simulink model "pwm_adc_sampling_timing"  (R2024b)
settings: Solver=FixedStepDiscrete  StartTime=0.0  StopTime=0  FixedStep=1  RelTol=1e-3
InitFcn:
  | model_file = get_param(bdroot, 'FileName');
  | model_dir = fileparts(model_file);
  | run(fullfile(model_dir, 'pwm_adc_sampling_params.m'));
values from neighbouring files (symbols this model uses):
  adc_fallback_ccr = pwm_half_arr    (= 2655)    [pwm_adc_sampling_params.m]
  adc_hold_last_on_fallback = 1    [pwm_adc_sampling_params.m]
  adc_margin_ccr = 140    [pwm_adc_sampling_params.m]
  adc_min_window_ccr = 320    [pwm_adc_sampling_params.m]
  adc_sample_max_ccr = pwm_arr - adc_margin_ccr    (= 5171)    [pwm_adc_sampling_params.m]
  adc_sample_min_ccr = adc_margin_ccr    (= 140)    [pwm_adc_sampling_params.m]
  pwm_arr = 5311    [pwm_adc_sampling_params.m]    (also in run_pwm_adc_sampling_timing_tests.m = local_param('pwm_arr'))
  pwm_half_arr = 2655    [pwm_adc_sampling_params.m]
  svpwm_max_ccr = pwm_arr - 20    (= 5291)    [pwm_adc_sampling_params.m]
  svpwm_min_ccr = 20    [pwm_adc_sampling_params.m]
  vbus = 24.0    (= 24)    [pwm_adc_sampling_params.m]
settings Model: Creator=10095  LastModifiedBy=10095

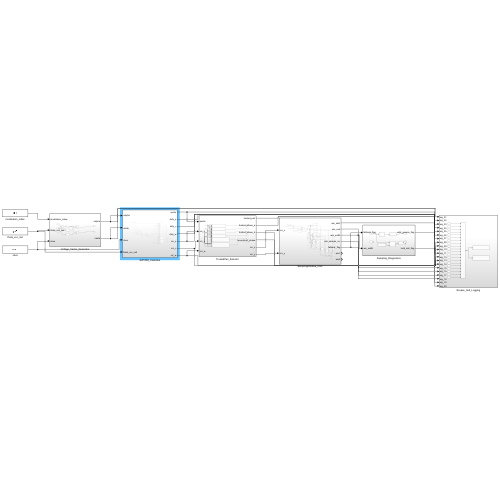
[thumbnail: Simulink's stored preview of the top-level diagram]
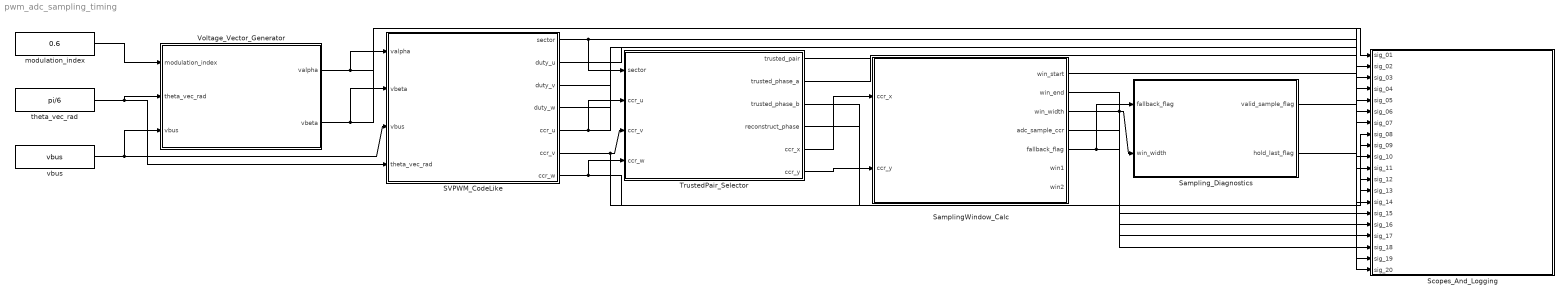
== system pwm_adc_sampling_timing ==
  SVPWM_CodeLike : Subsystem
  SamplingWindow_Calc : Subsystem
  Sampling_Diagnostics : Subsystem
  Scopes_And_Logging : Subsystem
  TrustedPair_Selector : Subsystem
  Voltage_Vector_Generator : Subsystem
  modulation_index : Constant  Value=0.6
  theta_vec_rad : Constant  Value=pi/6
  vbus : Constant  Value=vbus
  wires:
  modulation_index/1 -> Voltage_Vector_Generator/1(modulation_index)
  theta_vec_rad/1 -> Voltage_Vector_Generator/2(theta_vec_rad), SVPWM_CodeLike/4(theta_vec_rad)
  vbus/1 -> Voltage_Vector_Generator/3(vbus), SVPWM_CodeLike/3(vbus)
  Voltage_Vector_Generator/1(valpha) -> SVPWM_CodeLike/1(valpha), Scopes_And_Logging/1(sig_01)
  Voltage_Vector_Generator/2(vbeta) -> SVPWM_CodeLike/2(vbeta), Scopes_And_Logging/2(sig_02)
  SVPWM_CodeLike/1(sector) -> TrustedPair_Selector/1(sector), Scopes_And_Logging/3(sig_03)
  SVPWM_CodeLike/5(ccr_u) -> TrustedPair_Selector/2(ccr_u), Scopes_And_Logging/7(sig_07)
  SVPWM_CodeLike/6(ccr_v) -> TrustedPair_Selector/3(ccr_v), Scopes_And_Logging/8(sig_08)
  SVPWM_CodeLike/7(ccr_w) -> TrustedPair_Selector/4(ccr_w), Scopes_And_Logging/9(sig_09)
  TrustedPair_Selector/5(ccr_x) -> SamplingWindow_Calc/1(ccr_x)
  TrustedPair_Selector/6(ccr_y) -> SamplingWindow_Calc/2(ccr_y)
  SamplingWindow_Calc/5(fallback_flag) -> Sampling_Diagnostics/1(fallback_flag), Scopes_And_Logging/18(sig_18)
  SamplingWindow_Calc/3(win_width) -> Sampling_Diagnostics/2(win_width), Scopes_And_Logging/16(sig_16)
  SVPWM_CodeLike/2(duty_u) -> Scopes_And_Logging/4(sig_04)
  SVPWM_CodeLike/3(duty_v) -> Scopes_And_Logging/5(sig_05)
  SVPWM_CodeLike/4(duty_w) -> Scopes_And_Logging/6(sig_06)
  TrustedPair_Selector/1(trusted_pair) -> Scopes_And_Logging/10(sig_10)
  TrustedPair_Selector/2(trusted_phase_a) -> Scopes_And_Logging/11(sig_11)
  TrustedPair_Selector/3(trusted_phase_b) -> Scopes_And_Logging/12(sig_12)
  TrustedPair_Selector/4(reconstruct_phase) -> Scopes_And_Logging/13(sig_13)
  SamplingWindow_Calc/1(win_start) -> Scopes_And_Logging/14(sig_14)
  SamplingWindow_Calc/2(win_end) -> Scopes_And_Logging/15(sig_15)
  SamplingWindow_Calc/4(adc_sample_ccr) -> Scopes_And_Logging/17(sig_17)
  Sampling_Diagnostics/1(valid_sample_flag) -> Scopes_And_Logging/19(sig_19)
  Sampling_Diagnostics/2(hold_last_flag) -> Scopes_And_Logging/20(sig_20)

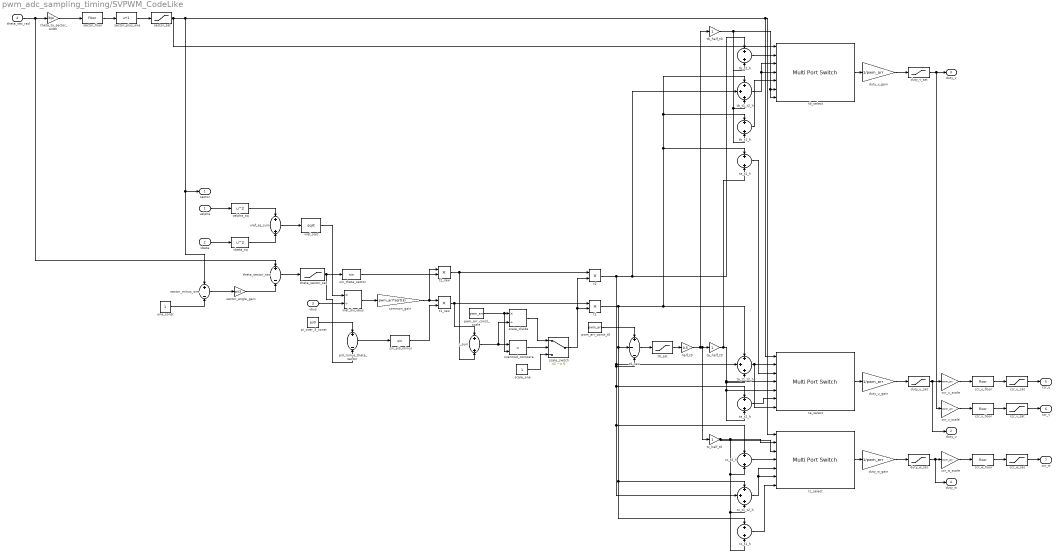
== system pwm_adc_sampling_timing/SVPWM_CodeLike ==
  valpha : Inport
  vbeta : Inport  Port=2
  vbus : Inport  Port=3
  theta_vec_rad : Inport  Port=4
  ccr_u_floor : Rounding
  ccr_u_sat : Saturate  UpperLimit=svpwm_max_ccr  LowerLimit=svpwm_min_ccr
  ccr_u_scale : Gain  Gain=pwm_arr
  ccr_v_floor : Rounding
  ccr_v_sat : Saturate  UpperLimit=svpwm_max_ccr  LowerLimit=svpwm_min_ccr
  ccr_v_scale : Gain  Gain=pwm_arr
  ccr_w_floor : Rounding
  ccr_w_sat : Saturate  UpperLimit=svpwm_max_ccr  LowerLimit=svpwm_min_ccr
  ccr_w_scale : Gain  Gain=pwm_arr
  common_gain : Gain  Gain=pwm_arr*sqrt(3)
  duty_u_gain : Gain  Gain=1/pwm_arr
  duty_u_sat : Saturate  UpperLimit=1  LowerLimit=0
  duty_v_gain : Gain  Gain=1/pwm_arr
  duty_v_sat : Saturate  UpperLimit=1  LowerLimit=0
  duty_w_gain : Gain  Gain=1/pwm_arr
  duty_w_sat : Saturate  UpperLimit=1  LowerLimit=0
  half_t0 : Gain  Gain=0.5
  one_const : Constant
  overmod_compare : RelationalOperator  Operator=>  OutDataTypeStr=boolean  RndMeth=Simplest  InputSameDT=off
  pi3_minus_theta_sector : Sum  Inputs=+-
  pi_over_3_const : Constant  Value=pi/3
  pwm_arr_const_scale : Constant  Value=pwm_arr
  pwm_arr_const_t0 : Constant  Value=pwm_arr
  scale_divide : Product  Inputs=*/
  scale_one : Constant
  scale_switch : Switch  Criteria=u2 ~= 0  SaturateOnIntegerOverflow=off  InputSameDT=off
  sector_angle_gain : Gain  Gain=pi/3
  sector_floor : Rounding
  sector_minus_one : Sum  Inputs=+-
  sector_plus_one : Bias  Bias=1  SaturateOnIntegerOverflow=off
  sector_sat : Saturate  UpperLimit=6  LowerLimit=1
  sin_pi3_minus : Trigonometry
  sin_theta_sector : Trigonometry
  t0_raw : Sum  Inputs=+--
  t0_sat : Saturate  UpperLimit=pwm_arr  LowerLimit=0
  t1 : Product
  t1_raw : Product
  t2 : Product
  t2_raw : Product
  t_sum : Sum
  ta_half_t0 : Gain
  ta_select : MultiPortSwitch  Inputs=6  SaturateOnIntegerOverflow=off  InputSameDT=off
  ta_t1_h : Sum
  ta_t1_t2_h : Sum  Inputs=+++
  ta_t2_h : Sum
  tb_half_t0 : Gain
  tb_select : MultiPortSwitch  Inputs=6  SaturateOnIntegerOverflow=off  InputSameDT=off
  tb_t1_h : Sum
  tb_t1_t2_h : Sum  Inputs=+++
  tb_t2_h : Sum
  tc_half_t0 : Gain
  tc_select : MultiPortSwitch  Inputs=6  SaturateOnIntegerOverflow=off  InputSameDT=off
  tc_t1_h : Sum
  tc_t1_t2_h : Sum  Inputs=+++
  tc_t2_h : Sum
  theta_sector_raw : Sum  Inputs=+-
  theta_sector_sat : Saturate  UpperLimit=pi/3  LowerLimit=0
  theta_to_sector_width : Gain  Gain=3/pi
  valpha_sq : Math  Operator=square
  vbeta_sq : Math  Operator=square
  vref_div_vbus : Product  Inputs=*/
  vref_sq_sum : Sum
  vref_sqrt : Math  Operator=sqrt
  sector : Outport
  duty_u : Outport  Port=2
  duty_v : Outport  Port=3
  duty_w : Outport  Port=4
  ccr_u : Outport  Port=5
  ccr_v : Outport  Port=6
  ccr_w : Outport  Port=7
  wires:
  theta_vec_rad/1 -> theta_to_sector_width/1, theta_sector_raw/1
  theta_to_sector_width/1 -> sector_floor/1
  sector_floor/1 -> sector_plus_one/1
  sector_sat/1 -> sector_minus_one/1, sector/1, ta_select/1, tc_select/1, tb_select/1
  sector_plus_one/1 -> sector_sat/1
  duty_v_gain/1 -> duty_v_sat/1
  one_const/1 -> sector_minus_one/2
  ta_t2_h/1 -> ta_select/6
  vbeta/1 -> vbeta_sq/1
  valpha/1 -> valpha_sq/1
  pi3_minus_theta_sector/1 -> sin_pi3_minus/1
  sector_minus_one/1 -> sector_angle_gain/1
  ccr_u_scale/1 -> ccr_u_floor/1
  valpha_sq/1 -> vref_sq_sum/1
  vbeta_sq/1 -> vref_sq_sum/2
  t0_sat/1 -> half_t0/1
  t0_raw/1 -> t0_sat/1
  sin_theta_sector/1 -> t2_raw/2
  sector_angle_gain/1 -> theta_sector_raw/2
  t1_raw/1 -> t1/1, t_sum/1
  vref_sq_sum/1 -> vref_sqrt/1
  ccr_v_floor/1 -> ccr_v_sat/1
  ta_half_t0/1 -> ta_t2_h/2, ta_select/5, ta_t1_t2_h/3, ta_select/4, ta_t1_h/2
  scale_switch/1 -> t1/2, t2/2
  theta_sector_raw/1 -> theta_sector_sat/1
  pwm_arr_const_scale/1 -> scale_divide/1, overmod_compare/2
  vref_sqrt/1 -> vref_div_vbus/1
  theta_sector_sat/1 -> pi3_minus_theta_sector/2, sin_theta_sector/1
  tc_select/1 -> duty_w_gain/1
  vbus/1 -> vref_div_vbus/2
  pi_over_3_const/1 -> pi3_minus_theta_sector/1
  vref_div_vbus/1 -> common_gain/1
  overmod_compare/1 -> scale_switch/2
  common_gain/1 -> t1_raw/1, t2_raw/1
  sin_pi3_minus/1 -> t1_raw/2
  ccr_w_sat/1 -> ccr_w/1
  t_sum/1 -> scale_divide/2, overmod_compare/1
  t2_raw/1 -> t_sum/2, t2/1
  scale_one/1 -> scale_switch/3
  scale_divide/1 -> scale_switch/1
  t2/1 -> tc_t2_h/1, tc_t1_t2_h/2, ta_t2_h/1, t0_raw/3, ta_t1_t2_h/2, tb_t2_h/1, tb_t1_t2_h/2
  tb_select/1 -> duty_v_gain/1
  t1/1 -> tc_t1_t2_h/1, tc_t1_h/1, t0_raw/2, tb_t1_h/1, tb_t1_t2_h/1, ta_t1_h/1, ta_t1_t2_h/1
  pwm_arr_const_t0/1 -> t0_raw/1
  ccr_w_scale/1 -> ccr_w_floor/1
  duty_w_sat/1 -> duty_w/1, ccr_w_scale/1
  duty_v_sat/1 -> duty_v/1, ccr_v_scale/1
  tb_t2_h/1 -> tb_select/2
  half_t0/1 -> tc_half_t0/1, ta_half_t0/1, tb_half_t0/1
  tb_half_t0/1 -> tb_t1_h/2, tb_t1_t2_h/3, tb_select/7, tb_select/6, tb_t2_h/2
  tc_half_t0/1 -> tc_t1_h/2, tc_t1_t2_h/3, tc_t2_h/2, tc_select/2, tc_select/3
  tb_t1_t2_h/1 -> tb_select/3, tb_select/4
  tb_t1_h/1 -> tb_select/5
  ta_t1_h/1 -> ta_select/3
  ta_t1_t2_h/1 -> ta_select/7, ta_select/2
  tc_t2_h/1 -> tc_select/4
  tc_t1_h/1 -> tc_select/7
  tc_t1_t2_h/1 -> tc_select/5, tc_select/6
  ta_select/1 -> duty_u_gain/1
  duty_u_gain/1 -> duty_u_sat/1
  duty_w_gain/1 -> duty_w_sat/1
  duty_u_sat/1 -> duty_u/1, ccr_u_scale/1
  ccr_v_scale/1 -> ccr_v_floor/1
  ccr_u_floor/1 -> ccr_u_sat/1
  ccr_w_floor/1 -> ccr_w_sat/1
  ccr_u_sat/1 -> ccr_u/1
  ccr_v_sat/1 -> ccr_v/1

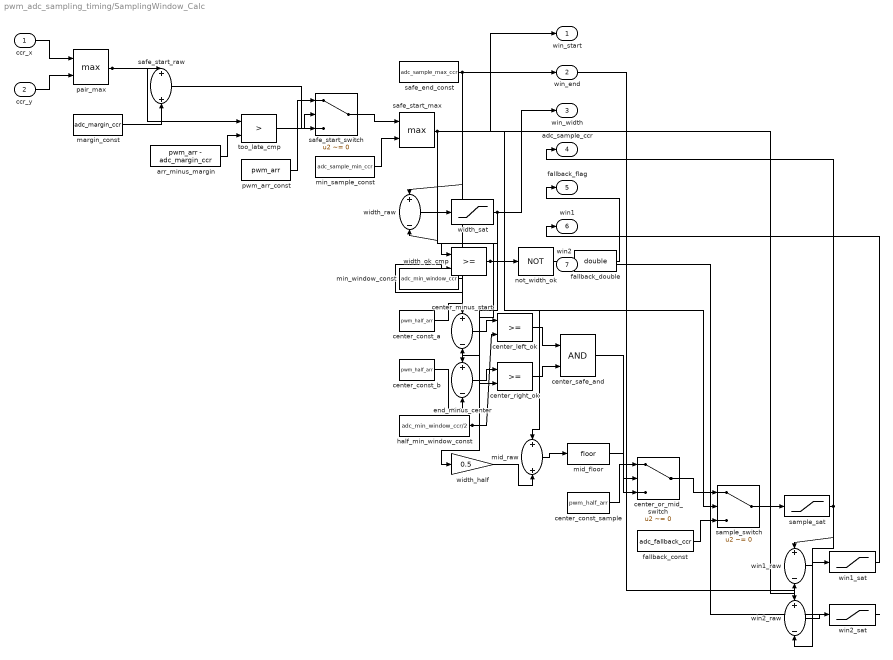
== system pwm_adc_sampling_timing/SamplingWindow_Calc ==
  ccr_x : Inport
  ccr_y : Inport  Port=2
  arr_minus_margin : Constant  Value=pwm_arr - adc_margin_ccr
  center_const_a : Constant  Value=pwm_half_arr
  center_const_b : Constant  Value=pwm_half_arr
  center_const_sample : Constant  Value=pwm_half_arr
  center_left_ok : RelationalOperator  OutDataTypeStr=boolean  RndMeth=Simplest  InputSameDT=off
  center_minus_start : Sum  Inputs=+-
  center_or_mid_switch : Switch  Criteria=u2 ~= 0  SaturateOnIntegerOverflow=off  InputSameDT=off
  center_right_ok : RelationalOperator  OutDataTypeStr=boolean  RndMeth=Simplest  InputSameDT=off
  center_safe_and : Logic  AllPortsSameDT=off  OutDataTypeStr=boolean
  end_minus_center : Sum  Inputs=+-
  fallback_const : Constant  Value=adc_fallback_ccr
  fallback_double : DataTypeConversion  OutDataTypeStr=double  SaturateOnIntegerOverflow=off  RndMeth=Floor
  half_min_window_const : Constant  Value=adc_min_window_ccr/2
  margin_const : Constant  Value=adc_margin_ccr
  mid_floor : Rounding
  mid_raw : Sum
  min_sample_const : Constant  Value=adc_sample_min_ccr
  min_window_const : Constant  Value=adc_min_window_ccr
  not_width_ok : Logic  Operator=NOT  AllPortsSameDT=off  OutDataTypeStr=boolean
  pair_max : MinMax  Function=max  Inputs=2
  pwm_arr_const : Constant  Value=pwm_arr
  safe_end_const : Constant  Value=adc_sample_max_ccr
  safe_start_max : MinMax  Function=max  Inputs=2
  safe_start_raw : Sum
  safe_start_switch : Switch  Criteria=u2 ~= 0  SaturateOnIntegerOverflow=off  InputSameDT=off
  sample_sat : Saturate  UpperLimit=svpwm_max_ccr  LowerLimit=svpwm_min_ccr
  sample_switch : Switch  Criteria=u2 ~= 0  SaturateOnIntegerOverflow=off  InputSameDT=off
  too_late_cmp : RelationalOperator  Operator=>  OutDataTypeStr=boolean  RndMeth=Simplest  InputSameDT=off
  width_half : Gain  Gain=0.5
  width_ok_cmp : RelationalOperator  OutDataTypeStr=boolean  RndMeth=Simplest  InputSameDT=off
  width_raw : Sum  Inputs=+-
  width_sat : Saturate  UpperLimit=pwm_arr  LowerLimit=0
  win1_raw : Sum  Inputs=+-
  win1_sat : Saturate  UpperLimit=pwm_arr  LowerLimit=0
  win2_raw : Sum  Inputs=+-
  win2_sat : Saturate  UpperLimit=pwm_arr  LowerLimit=0
  win_start : Outport
  win_end : Outport  Port=2
  win_width : Outport  Port=3
  adc_sample_ccr : Outport  Port=4
  fallback_flag : Outport  Port=5
  win1 : Outport  Port=6
  win2 : Outport  Port=7
  wires:
  ccr_x/1 -> pair_max/1
  ccr_y/1 -> pair_max/2
  pair_max/1 -> safe_start_raw/1, too_late_cmp/1
  margin_const/1 -> safe_start_raw/2
  arr_minus_margin/1 -> too_late_cmp/2
  pwm_arr_const/1 -> safe_start_switch/1
  too_late_cmp/1 -> safe_start_switch/2
  safe_start_raw/1 -> safe_start_switch/3
  safe_start_switch/1 -> safe_start_max/1
  min_sample_const/1 -> safe_start_max/2
  safe_start_max/1 -> win_start/1, width_raw/2, center_minus_start/2, mid_raw/1, win1_raw/2
  safe_end_const/1 -> win_end/1, width_raw/1, end_minus_center/1, win2_raw/1
  width_raw/1 -> width_sat/1
  width_sat/1 -> win_width/1, width_ok_cmp/1, width_half/1
  min_window_const/1 -> width_ok_cmp/2
  width_ok_cmp/1 -> not_width_ok/1, sample_switch/2
  not_width_ok/1 -> fallback_double/1
  fallback_double/1 -> fallback_flag/1
  center_const_a/1 -> center_minus_start/1
  center_const_b/1 -> end_minus_center/2
  center_minus_start/1 -> center_left_ok/1
  half_min_window_const/1 -> center_left_ok/2, center_right_ok/2
  end_minus_center/1 -> center_right_ok/1
  center_left_ok/1 -> center_safe_and/1
  center_right_ok/1 -> center_safe_and/2
  width_half/1 -> mid_raw/2
  mid_raw/1 -> mid_floor/1
  center_const_sample/1 -> center_or_mid_switch/1
  center_safe_and/1 -> center_or_mid_switch/2
  mid_floor/1 -> center_or_mid_switch/3
  center_or_mid_switch/1 -> sample_switch/1
  fallback_const/1 -> sample_switch/3
  sample_switch/1 -> sample_sat/1
  sample_sat/1 -> adc_sample_ccr/1, win1_raw/1, win2_raw/2
  win1_raw/1 -> win1_sat/1
  win1_sat/1 -> win1/1
  win2_raw/1 -> win2_sat/1
  win2_sat/1 -> win2/1

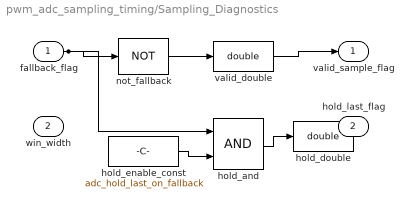
== system pwm_adc_sampling_timing/Sampling_Diagnostics ==
  fallback_flag : Inport
  win_width : Inport  Port=2
  hold_and : Logic  AllPortsSameDT=off  OutDataTypeStr=boolean
  hold_double : DataTypeConversion  OutDataTypeStr=double  SaturateOnIntegerOverflow=off  RndMeth=Floor
  hold_enable_const : Constant  Value=adc_hold_last_on_fallback
  not_fallback : Logic  Operator=NOT  AllPortsSameDT=off  OutDataTypeStr=boolean
  valid_double : DataTypeConversion  OutDataTypeStr=double  SaturateOnIntegerOverflow=off  RndMeth=Floor
  valid_sample_flag : Outport
  hold_last_flag : Outport  Port=2
  wires:
  fallback_flag/1 -> not_fallback/1, hold_and/1
  not_fallback/1 -> valid_double/1
  valid_double/1 -> valid_sample_flag/1
  hold_enable_const/1 -> hold_and/2
  hold_and/1 -> hold_double/1
  hold_double/1 -> hold_last_flag/1

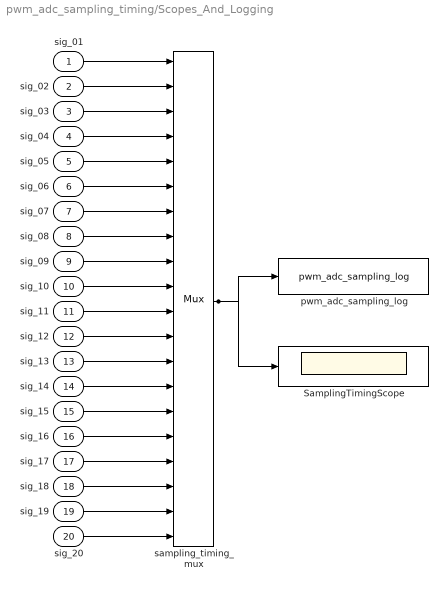
== system pwm_adc_sampling_timing/Scopes_And_Logging ==
  sig_01 : Inport
  sig_02 : Inport  Port=2
  sig_03 : Inport  Port=3
  sig_04 : Inport  Port=4
  sig_05 : Inport  Port=5
  sig_06 : Inport  Port=6
  sig_07 : Inport  Port=7
  sig_08 : Inport  Port=8
  sig_09 : Inport  Port=9
  sig_10 : Inport  Port=10
  sig_11 : Inport  Port=11
  sig_12 : Inport  Port=12
  sig_13 : Inport  Port=13
  sig_14 : Inport  Port=14
  sig_15 : Inport  Port=15
  sig_16 : Inport  Port=16
  sig_17 : Inport  Port=17
  sig_18 : Inport  Port=18
  sig_19 : Inport  Port=19
  sig_20 : Inport  Port=20
  SamplingTimingScope : Scope
  pwm_adc_sampling_log : ToWorkspace  VariableName=pwm_adc_sampling_log  SampleTime=-1
  sampling_timing_mux : Mux  Inputs=20
  wires:
  sig_01/1 -> sampling_timing_mux/1
  sig_02/1 -> sampling_timing_mux/2
  sig_03/1 -> sampling_timing_mux/3
  sig_04/1 -> sampling_timing_mux/4
  sig_05/1 -> sampling_timing_mux/5
  sig_06/1 -> sampling_timing_mux/6
  sig_07/1 -> sampling_timing_mux/7
  sig_08/1 -> sampling_timing_mux/8
  sig_09/1 -> sampling_timing_mux/9
  sig_10/1 -> sampling_timing_mux/10
  sig_11/1 -> sampling_timing_mux/11
  sig_12/1 -> sampling_timing_mux/12
  sig_13/1 -> sampling_timing_mux/13
  sig_14/1 -> sampling_timing_mux/14
  sig_15/1 -> sampling_timing_mux/15
  sig_16/1 -> sampling_timing_mux/16
  sig_17/1 -> sampling_timing_mux/17
  sig_18/1 -> sampling_timing_mux/18
  sig_19/1 -> sampling_timing_mux/19
  sig_20/1 -> sampling_timing_mux/20
  sampling_timing_mux/1 -> pwm_adc_sampling_log/1, SamplingTimingScope/1

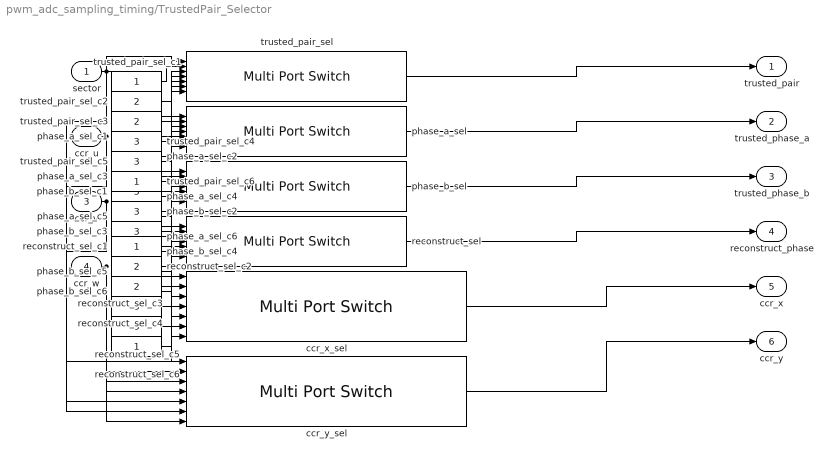
== system pwm_adc_sampling_timing/TrustedPair_Selector ==
  sector : Inport
  ccr_u : Inport  Port=2
  ccr_v : Inport  Port=3
  ccr_w : Inport  Port=4
  ccr_x_sel : MultiPortSwitch  Inputs=6  SaturateOnIntegerOverflow=off  InputSameDT=off
  ccr_y_sel : MultiPortSwitch  Inputs=6  SaturateOnIntegerOverflow=off  InputSameDT=off
  phase_a_sel : MultiPortSwitch  Inputs=6  SaturateOnIntegerOverflow=off  InputSameDT=off
  phase_a_sel_c1 : Constant  Value=2
  phase_a_sel_c{2..5} (4 alike) : Constant
  phase_a_sel_c6 : Constant  Value=2
  phase_b_sel : MultiPortSwitch  Inputs=6  SaturateOnIntegerOverflow=off  InputSameDT=off
  phase_b_sel_c{1..3,6} (4 alike) : Constant  Value=3
  phase_b_sel_c4 : Constant  Value=2
  phase_b_sel_c5 : Constant  Value=2
  reconstruct_sel : MultiPortSwitch  Inputs=6  SaturateOnIntegerOverflow=off  InputSameDT=off
  reconstruct_sel_c1 : Constant
  reconstruct_sel_c2 : Constant  Value=2
  reconstruct_sel_c3 : Constant  Value=2
  reconstruct_sel_c4 : Constant  Value=3
  reconstruct_sel_c5 : Constant  Value=3
  reconstruct_sel_c6 : Constant
  trusted_pair_sel : MultiPortSwitch  Inputs=6  SaturateOnIntegerOverflow=off  InputSameDT=off
  trusted_pair_sel_c1 : Constant
  trusted_pair_sel_c2 : Constant  Value=2
  trusted_pair_sel_c3 : Constant  Value=2
  trusted_pair_sel_c4 : Constant  Value=3
  trusted_pair_sel_c5 : Constant  Value=3
  trusted_pair_sel_c6 : Constant
  trusted_pair : Outport
  trusted_phase_a : Outport  Port=2
  trusted_phase_b : Outport  Port=3
  reconstruct_phase : Outport  Port=4
  ccr_x : Outport  Port=5
  ccr_y : Outport  Port=6
  wires:
  trusted_pair_sel_c1/1 -> trusted_pair_sel/2
  trusted_pair_sel_c2/1 -> trusted_pair_sel/3
  trusted_pair_sel_c3/1 -> trusted_pair_sel/4
  trusted_pair_sel_c4/1 -> trusted_pair_sel/5
  trusted_pair_sel_c5/1 -> trusted_pair_sel/6
  trusted_pair_sel_c6/1 -> trusted_pair_sel/7
  phase_a_sel_c1/1 -> phase_a_sel/2
  phase_a_sel_c2/1 -> phase_a_sel/3
  phase_a_sel_c3/1 -> phase_a_sel/4
  phase_a_sel_c4/1 -> phase_a_sel/5
  phase_a_sel_c5/1 -> phase_a_sel/6
  phase_a_sel_c6/1 -> phase_a_sel/7
  phase_b_sel_c1/1 -> phase_b_sel/2
  phase_b_sel_c2/1 -> phase_b_sel/3
  phase_b_sel_c3/1 -> phase_b_sel/4
  phase_b_sel_c4/1 -> phase_b_sel/5
  phase_b_sel_c5/1 -> phase_b_sel/6
  phase_b_sel_c6/1 -> phase_b_sel/7
  reconstruct_sel_c1/1 -> reconstruct_sel/2
  reconstruct_sel_c2/1 -> reconstruct_sel/3
  reconstruct_sel_c3/1 -> reconstruct_sel/4
  reconstruct_sel_c4/1 -> reconstruct_sel/5
  reconstruct_sel_c5/1 -> reconstruct_sel/6
  reconstruct_sel_c6/1 -> reconstruct_sel/7
  ccr_v/1 -> ccr_x_sel/2, ccr_x_sel/7, ccr_y_sel/5, ccr_y_sel/6
  ccr_u/1 -> ccr_x_sel/3, ccr_x_sel/4, ccr_x_sel/5, ccr_x_sel/6
  ccr_w/1 -> ccr_y_sel/2, ccr_y_sel/3, ccr_y_sel/4, ccr_y_sel/7
  sector/1 -> trusted_pair_sel/1, phase_a_sel/1, phase_b_sel/1, reconstruct_sel/1, ccr_x_sel/1, ccr_y_sel/1
  trusted_pair_sel/1 -> trusted_pair/1
  phase_a_sel/1 -> trusted_phase_a/1
  phase_b_sel/1 -> trusted_phase_b/1
  reconstruct_sel/1 -> reconstruct_phase/1
  ccr_x_sel/1 -> ccr_x/1
  ccr_y_sel/1 -> ccr_y/1

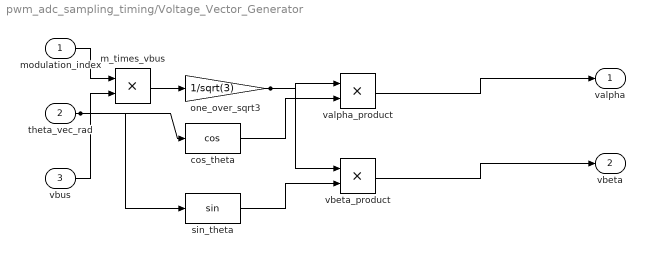
== system pwm_adc_sampling_timing/Voltage_Vector_Generator ==
  modulation_index : Inport
  theta_vec_rad : Inport  Port=2
  vbus : Inport  Port=3
  cos_theta : Trigonometry  Operator=cos
  m_times_vbus : Product
  one_over_sqrt3 : Gain  Gain=1/sqrt(3)
  sin_theta : Trigonometry
  valpha_product : Product
  vbeta_product : Product
  valpha : Outport
  vbeta : Outport  Port=2
  wires:
  modulation_index/1 -> m_times_vbus/1
  vbus/1 -> m_times_vbus/2
  m_times_vbus/1 -> one_over_sqrt3/1
  theta_vec_rad/1 -> cos_theta/1, sin_theta/1
  one_over_sqrt3/1 -> valpha_product/1, vbeta_product/1
  cos_theta/1 -> valpha_product/2
  sin_theta/1 -> vbeta_product/2
  valpha_product/1 -> valpha/1
  vbeta_product/1 -> vbeta/1
